simulink model "zad3_model2"  (R2017a)
settings: Solver=VariableStepAuto  StartTime=0.0  StopTime=10.0  RelTol=1e-3
values from neighbouring files (symbols this model uses):
  K = acker(A2, B2, [z z z])    [zad3a.m]    (also in zad3b.m = acker(A2, B2, [z1 z2 z2]); zad3max.m; zad4.m = acker(Ap, Bp, [0.6 0.4 0.4]))
  Tp = 0.1    [zad3a.m]    (also in zad3b.m; zad3max.m; zad4.m)
settings Model: Creator=Rajtek  LastModifiedBy=Rajtek

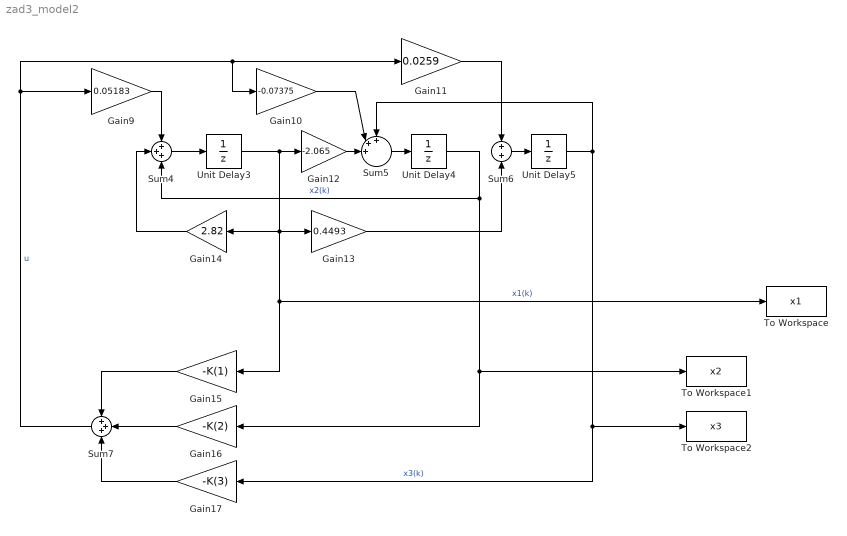
== system zad3_model2 ==
  Gain10 : Gain  Gain=-0.07375
  Gain11 : Gain  Gain=0.0259
  Gain12 : Gain  Gain=-2.065
  Gain13 : Gain  Gain=0.4493
  Gain14 : Gain  Gain=2.82
  Gain15 : Gain  Gain=-K(1)
  Gain16 : Gain  Gain=-K(2)
  Gain17 : Gain  Gain=-K(3)
  Gain9 : Gain  Gain=0.05183
  Sum4 : Sum  Inputs=+++
  Sum5 : Sum  Inputs=+++||
  Sum6 : Sum  Inputs=+|+
  Sum7 : Sum  Inputs=+++
  To Workspace : ToWorkspace  VariableName=x1  SaveFormat=Timeseries  SampleTime=-1
  To Workspace1 : ToWorkspace  VariableName=x2  SaveFormat=Timeseries  SampleTime=-1
  To Workspace2 : ToWorkspace  VariableName=x3  SaveFormat=Timeseries  SampleTime=-1
  Unit Delay3 : UnitDelay  InitialCondition=1  SampleTime=Tp
  Unit Delay4 : UnitDelay  InitialCondition=-2  SampleTime=Tp
  Unit Delay5 : UnitDelay  InitialCondition=2  SampleTime=Tp
  wires:
  Gain12/1 -> Sum5/3
  Gain13/1 -> Sum6/2
  Gain16/1 -> Sum7/2
  Gain14/1 -> Sum4/2
  Gain11/1 -> Sum6/1
  Sum5/1 -> Unit Delay4/1
  Unit Delay5/1 -> Gain17/1, To Workspace2/1, Sum5/1  "x3(k)"
  Gain17/1 -> Sum7/3
  Unit Delay4/1 -> Gain16/1, To Workspace1/1, Sum4/3  "x2(k)"
  Gain15/1 -> Sum7/1
  Sum7/1 -> Gain9/1, Gain11/1, Gain10/1  "u"
  Gain9/1 -> Sum4/1
  Gain10/1 -> Sum5/2
  Unit Delay3/1 -> Gain15/1, To Workspace/1, Gain13/1, Gain14/1, Gain12/1  "x1(k)"
  Sum4/1 -> Unit Delay3/1
  Sum6/1 -> Unit Delay5/1
